simulink model "Adblue_Level_and_heater"  (R2019a)
settings: Solver=FixedStepDiscrete  StartTime=0.0  StopTime=10.0  FixedStep=1  RelTol=1e-3
settings Model: DataDictionary=Adblue_Level_and_heater_DD.sldd  Creator=Kore  LastModifiedBy=Kore
settings ConfigComp: CovEnable=on  RecordCoverage=on  CovMetricSettings=dcmw  CovHtmlReporting=on  CovModelRefEnable=on  DVMode=DesignErrorDetection  DVBlockReplacement=on  DVModelCoverageObjectives=MCDC  DVTestSuiteOptimization=Auto  DVDetectDeadLogic=on  DVDetectActiveLogic=on  DVDetectOutOfBounds=on  DVSaveHarnessModel=on  DVSaveReport=on  DVReportPDFFormat=on  DVRebuildModelRepresentation=Always

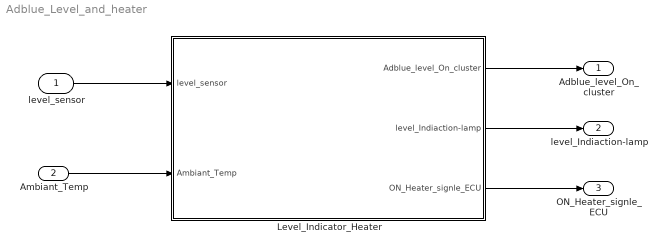
== system Adblue_Level_and_heater ==
  level_sensor : Inport
  Ambiant_Temp : Inport  Port=2
  Level_Indicator_Heater : Subsystem
  Adblue_level_On_cluster : Outport
  level_Indiaction-lamp : Outport  Port=2
  ON_Heater_signle_ECU : Outport  Port=3
  wires:
  Ambiant_Temp/1 -> Level_Indicator_Heater/2(Ambiant_Temp)
  level_sensor/1 -> Level_Indicator_Heater/1(level_sensor)
  Level_Indicator_Heater/1(Adblue_level_On_cluster) -> Adblue_level_On_cluster/1
  Level_Indicator_Heater/2(level_Indiaction-lamp) -> level_Indiaction-lamp/1
  Level_Indicator_Heater/3(ON_Heater_signle_ECU) -> ON_Heater_signle_ECU/1

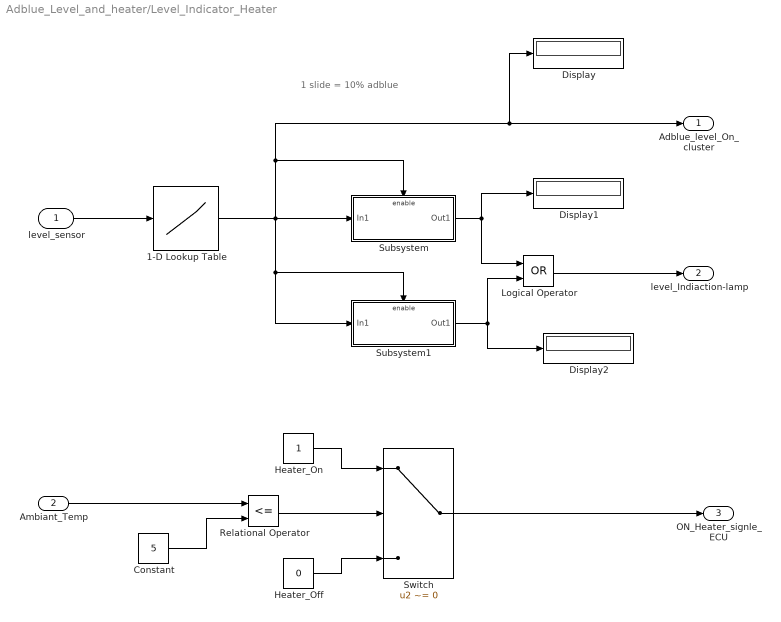
== system Adblue_Level_and_heater/Level_Indicator_Heater ==
  note: 1 slide = 10% adblue
  level_sensor : Inport
  Ambiant_Temp : Inport  Port=2
  1-D Lookup Table : Lookup_n-D  NumberOfTableDimensions=1  BreakpointsForDimension1=[0:10:100]  Table=[0:1:10]  InternalRulePriority=Speed  RndMeth=Simplest  InputSameDT=on
  Constant : Constant  Value=5
  Display : Display
  Display1 : Display
  Display2 : Display
  Heater_Off : Constant  Value=0
  Heater_On : Constant
  Logical Operator : Logic  Operator=OR  AllPortsSameDT=off  OutDataTypeStr=boolean
  Relational Operator : RelationalOperator  Operator=<=  OutDataTypeStr=boolean  RndMeth=Simplest
  Subsystem : Subsystem
  Subsystem1 : Subsystem
  Switch : Switch  Criteria=u2 ~= 0
  Adblue_level_On_cluster : Outport
  level_Indiaction-lamp : Outport  Port=2
  ON_Heater_signle_ECU : Outport  Port=3
  wires:
  level_sensor/1 -> 1-D Lookup Table/1
  Subsystem1/1(Out1) -> Logical Operator/2, Display2/1
  Logical Operator/1 -> level_Indiaction-lamp/1
  1-D Lookup Table/1 -> Adblue_level_On_cluster/1, Display/1, Subsystem/Enable, Subsystem1/1(In1), Subsystem1/Enable, Subsystem/1(In1)
  Subsystem/1(Out1) -> Display1/1, Logical Operator/1
  Constant/1 -> Relational Operator/2
  Relational Operator/1 -> Switch/2
  Ambiant_Temp/1 -> Relational Operator/1
  Heater_On/1 -> Switch/1
  Heater_Off/1 -> Switch/3
  Switch/1 -> ON_Heater_signle_ECU/1

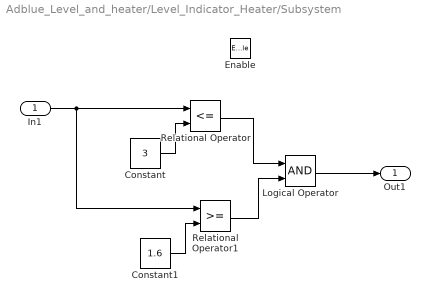
== system Adblue_Level_and_heater/Level_Indicator_Heater/Subsystem ==
  In1 : Inport
  Enable : EnablePort  StatesWhenEnabling=reset
  Constant : Constant  Value=3
  Constant1 : Constant  Value=1.6
  Logical Operator : Logic  AllPortsSameDT=off  OutDataTypeStr=boolean
  Relational Operator : RelationalOperator  Operator=<=  OutDataTypeStr=boolean  RndMeth=Simplest
  Relational Operator1 : RelationalOperator  OutDataTypeStr=boolean  RndMeth=Simplest
  Out1 : Outport
  wires:
  Constant/1 -> Relational Operator/2
  Constant1/1 -> Relational Operator1/2
  In1/1 -> Relational Operator1/1, Relational Operator/1
  Relational Operator/1 -> Logical Operator/1
  Relational Operator1/1 -> Logical Operator/2
  Logical Operator/1 -> Out1/1

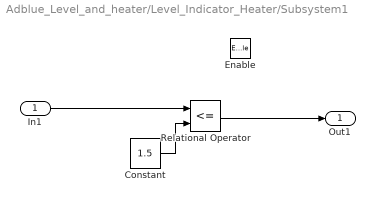
== system Adblue_Level_and_heater/Level_Indicator_Heater/Subsystem1 ==
  In1 : Inport
  Enable : EnablePort  StatesWhenEnabling=reset
  Constant : Constant  Value=1.5
  Relational Operator : RelationalOperator  Operator=<=  OutDataTypeStr=boolean  RndMeth=Simplest
  Out1 : Outport
  wires:
  Relational Operator/1 -> Out1/1
  In1/1 -> Relational Operator/1
  Constant/1 -> Relational Operator/2
